simulink model "bike_model_cl"  (R2022b)
settings: Solver=FixedStepAuto  StartTime=0.0  StopTime=20  FixedStep=0.01  RelTol=1e-3
undefined symbols (not defined in the file): gearboxRatio, massTotal_kg, wheelBase_m, wheelBaseRear_m, wheelRadius_m
libraries: autolibshared x3, simulink_extras x2, slpidlib x1
settings Model: Creator=LinF  LastModifiedBy=maxfa
settings SolverCC: ConcurrentTasks=on  PositivePriorityOrder=on
settings OptimizationCC: BlockReduction=off  OptimizeBlockIOStorage=off  BufferReuse=off
settings DebuggingCC: TasksWithSamePriorityMsg=none
settings HardwareCC: ProdBitPerLong=64  ProdLongLongMode=on  ProdHWDeviceType=Intel->x86-64 (Linux 64)
settings RTWCC: Description=Simulink Real-Time  SystemTargetFile=slrealtime.tlc  TemplateMakefile=slrealtime_default_tmf  Toolchain=Simulink Real-Time Toolchain  BuildConfiguration=Faster Runs  CodeExecutionProfiling=on  TargetLang=C++

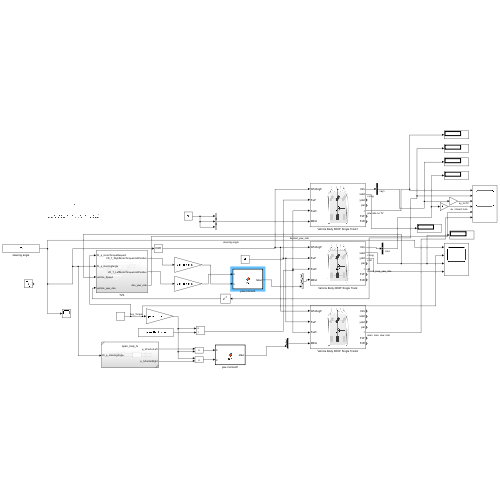
[thumbnail: Simulink's stored preview of the top-level diagram]
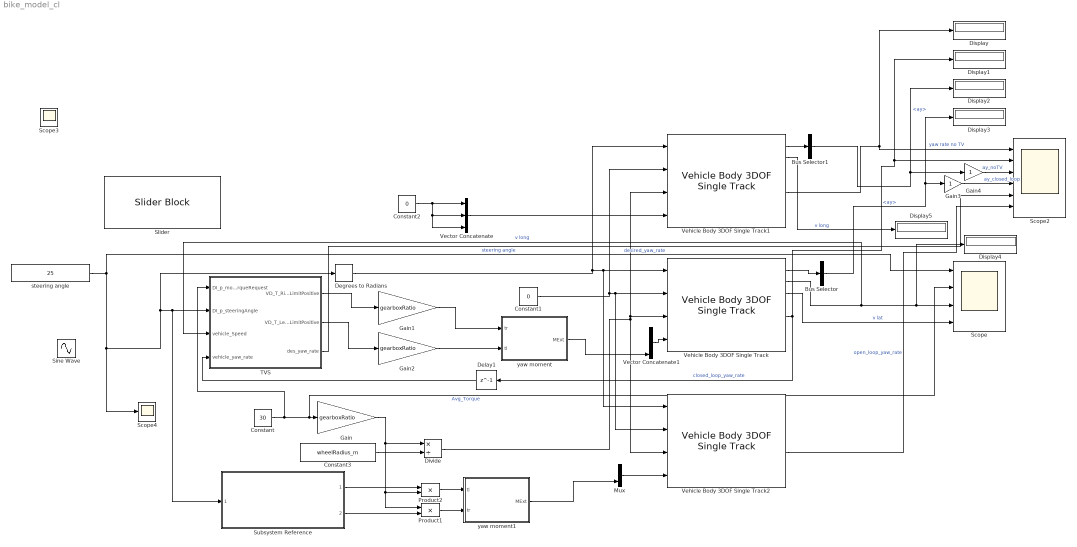
== system bike_model_cl ==
  Bus Selector : BusSelector  OutputSignals=BdyFrm.Cg.Acc.ay
  Bus Selector1 : BusSelector  OutputSignals=BdyFrm.Cg.Acc.ay
  Constant : Constant  Value=30
  Constant1 : Constant  Value=0
  Constant2 : Constant  Value=0
  Constant3 : Constant  Value=wheelRadius_m
  Degrees to Radians : simulink_extras/Transformations/Degrees to Radians
  Delay1 : Delay  DelayLength=1
  Display{,1..5} (6 alike) : Display
  Divide : Product  Inputs=*/
  Gain : Gain  Gain=gearboxRatio
  Gain1 : Gain  Gain=gearboxRatio
  Gain2 : Gain  Gain=gearboxRatio
  Gain3 : Gain
  Gain4 : Gain
  Mux : Mux  Inputs=3
  Product1 : Product
  Product2 : Product
  Scope : Scope  NumInputPorts=4
  Scope2 : Scope  NumInputPorts=6
  Scope4 : Scope
  Sine Wave : Sin  Amplitude=25  SampleTime=0
  Slider : SliderBlock  ScaleMin=-25  ScaleMax=25
  Subsystem Reference : Subsystem  ReferencedSubsystem=open_loop_tv
  TVS : Subsystem
  Vector Concatenate : Concatenate  NumInputs=3
  Vector Concatenate1 : Concatenate  NumInputs=3
  Vehicle Body 3DOF Single Track : autolibshared/Vehicle Body 3DOF Single Track  trackMode=Single (bicycle)  inputMode=External longitudinal forces  frontSteerMode=on  rearSteerMode=off  windMode=off  muMode=off  extFMode=off  extMMode=on  htchFMode=off  htchMMode=off  extXo=off  extpsio=off  extxdoto=off  extro=off  extYo=off  extTamb=off  extydoto=off  aMode=2  NF=2  NR=2  m=massTotal_kg  a=wheelBaseFront_m  b=wheelBaseRear_m  h=cgHeight_m  dh=1  hh=0.2  X_o=0  xdot_o=0  CalphaMode=off  sigmaMode=off  d=0  hl=0  w=[1.4,1.4]  Cy_f=CyFront_N_per_Rad  Cy_r=CyRear_N_per_Rad  sigma_f=.1  sigma_r=.1  alpha_f_brk=[-.1 .1]  Cy_f_data=[-9e3 9e3]  alpha_r_brk=[-.1 .1]  Cy_r_data=[-9e3 9e3]  Y_o=0  ydot_o=0  Izz=yawInertia_kg_per_mSqrd  psi_o=0  r_o=0  Af=dragArea_mSqrd  Cd=Cd  Cl=Cl  Cpm=.1  beta_w=[0 0.01:0.01:0.3]  Cs=[0 0.01:0.01:0.3]  Cym=[0 1e-6:0.01:0.3]  Pabs=101325  Tair=273  g=9.81  mu=1  xdot_tol=.01  Fznom=5000  Fxtire_sat=7e4  Fytire_sat=7e4  longOff=0  latOff=0  vertOff=0  wrapAng=off
  Vehicle Body 3DOF Single Track1 : autolibshared/Vehicle Body 3DOF Single Track  trackMode=Single (bicycle)  inputMode=External longitudinal forces  frontSteerMode=on  rearSteerMode=off  windMode=off  muMode=off  extFMode=off  extMMode=on  htchFMode=off  htchMMode=off  extXo=off  extpsio=off  extxdoto=off  extro=off  extYo=off  extTamb=off  extydoto=off  aMode=2  NF=2  NR=2  m=massTotal_kg  a=wheelBaseFront_m  b=wheelBaseRear_m  h=cgHeight_m  dh=1  hh=0.2  X_o=0  xdot_o=0  CalphaMode=off  sigmaMode=off  d=0  hl=0  w=[1.4,1.4]  Cy_f=CyFront_N_per_Rad  Cy_r=CyRear_N_per_Rad  sigma_f=.1  sigma_r=.1  alpha_f_brk=[-.1 .1]  Cy_f_data=[-9e3 9e3]  alpha_r_brk=[-.1 .1]  Cy_r_data=[-9e3 9e3]  Y_o=0  ydot_o=0  Izz=yawInertia_kg_per_mSqrd  psi_o=0  r_o=0  Af=dragArea_mSqrd  Cd=Cd  Cl=Cl  Cpm=.1  beta_w=[0 0.01:0.01:0.3]  Cs=[0 0.01:0.01:0.3]  Cym=[0 1e-6:0.01:0.3]  Pabs=101325  Tair=273  g=9.81  mu=1  xdot_tol=.01  Fznom=5000  Fxtire_sat=7e4  Fytire_sat=7e4  longOff=0  latOff=0  vertOff=0  wrapAng=off
  Vehicle Body 3DOF Single Track2 : autolibshared/Vehicle Body 3DOF Single Track  trackMode=Single (bicycle)  inputMode=External longitudinal forces  frontSteerMode=on  rearSteerMode=off  windMode=off  muMode=off  extFMode=off  extMMode=on  htchFMode=off  htchMMode=off  extXo=off  extpsio=off  extxdoto=off  extro=off  extYo=off  extTamb=off  extydoto=off  aMode=2  NF=2  NR=2  m=massTotal_kg  a=wheelBaseFront_m  b=wheelBaseRear_m  h=cgHeight_m  dh=1  hh=0.2  X_o=0  xdot_o=0  CalphaMode=off  sigmaMode=off  d=0  hl=0  w=[1.4,1.4]  Cy_f=CyFront_N_per_Rad  Cy_r=CyRear_N_per_Rad  sigma_f=.1  sigma_r=.1  alpha_f_brk=[-.1 .1]  Cy_f_data=[-9e3 9e3]  alpha_r_brk=[-.1 .1]  Cy_r_data=[-9e3 9e3]  Y_o=0  ydot_o=0  Izz=yawInertia_kg_per_mSqrd  psi_o=0  r_o=0  Af=dragArea_mSqrd  Cd=Cd  Cl=Cl  Cpm=.1  beta_w=[0 0.01:0.01:0.3]  Cs=[0 0.01:0.01:0.3]  Cym=[0 1e-6:0.01:0.3]  Pabs=101325  Tair=273  g=9.81  mu=1  xdot_tol=.01  Fznom=5000  Fxtire_sat=7e4  Fytire_sat=7e4  longOff=0  latOff=0  vertOff=0  wrapAng=off
  steering angle : Constant  Value=25
  yaw moment : MATLAB Function  TreatAsAtomicUnit=on
  yaw moment1 : MATLAB Function  TreatAsAtomicUnit=on
  Scope3 : Scope
  wires:
  Vehicle Body 3DOF Single Track/1 -> Bus Selector/1
  Vehicle Body 3DOF Single Track/3 -> Scope/4  "v lat"
  Vehicle Body 3DOF Single Track/2 -> TVS/3(vehicle_Speed), Display4/1, Scope/3  "v long"
  Vehicle Body 3DOF Single Track/5 -> Scope2/2, Display1/1, Delay1/1  "closed_loop_yaw_rate"
  Constant/1 -> TVS/1(DI_p_motorTorqueRequest), Scope/2, Gain/1  "Avg_Torque"
  Degrees to Radians/1 -> Vehicle Body 3DOF Single Track2/1, Vehicle Body 3DOF Single Track/1, Vehicle Body 3DOF Single Track1/1
  yaw moment/1(MExt) -> Vector Concatenate1/3
  steering angle/1 -> Scope/1, Scope4/1, Degrees to Radians/1, Subsystem Reference/1, TVS/2(DI_p_steeringAngle)  "steering angle"
  Vector Concatenate/1 -> Vehicle Body 3DOF Single Track1/4
  Vehicle Body 3DOF Single Track1/5 -> Display/1, Scope2/1  "yaw rate no TV"
  Constant2/1 -> Vector Concatenate/3, Vector Concatenate/2, Vector Concatenate/1
  Constant1/1 -> Vehicle Body 3DOF Single Track2/2, Vehicle Body 3DOF Single Track/2, Vehicle Body 3DOF Single Track1/2
  Constant3/1 -> Divide/2
  Divide/1 -> Vehicle Body 3DOF Single Track/3, Vehicle Body 3DOF Single Track1/3, Vehicle Body 3DOF Single Track2/3
  Vehicle Body 3DOF Single Track1/1 -> Bus Selector1/1
  Bus Selector1/1 -> Display2/1, Gain4/1  "<ay>"
  Bus Selector/1 -> Gain3/1, Display3/1  "<ay>"
  Gain/1 -> Product2/2, Product1/1, Divide/1
  Vehicle Body 3DOF Single Track1/2 -> Display5/1  "v long"
  TVS/1(VD_T_RightMotorTorqueLimitPositive) -> Gain1/1
  TVS/2(VD_T_LeftMotorTorqueLimitPositive) -> Gain2/1
  Delay1/1 -> TVS/4(vehicle_yaw_rate)
  Vector Concatenate1/1 -> Vehicle Body 3DOF Single Track/4
  TVS/3(des_yaw_rate) -> Scope2/5  "desired_yaw_rate"
  Gain1/1 -> yaw moment/1(tr)
  Gain2/1 -> yaw moment/2(tl)
  Product2/1 -> yaw moment1/1(tl)
  Product1/1 -> yaw moment1/2(tr)
  Subsystem Reference/1 -> Product2/1
  Subsystem Reference/2 -> Product1/2
  Vehicle Body 3DOF Single Track2/5 -> Scope2/6  "open_loop_yaw_rate"
  Mux/1 -> Vehicle Body 3DOF Single Track2/4
  yaw moment1/1(MExt) -> Mux/3
  Gain3/1 -> Scope2/4  "ay_closed_loop"
  Gain4/1 -> Scope2/3  "ay_noTV"

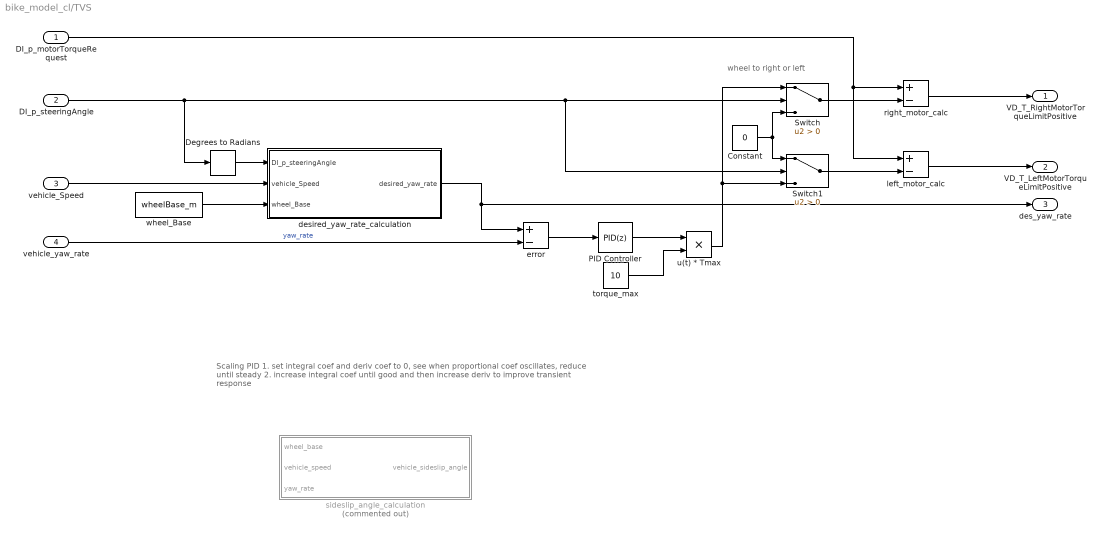
== system bike_model_cl/TVS ==
  note: wheel to right or left
  note: Scaling PID
      | 1. set integral coef and deriv coef to 0, see when proportional coef oscillates, reduce until steady
      | 2. increase integral coef until good and then increase deriv to improve transient response
  DI_p_motorTorqueRequest : Inport
  DI_p_steeringAngle : Inport  Port=2
  vehicle_Speed : Inport  Port=3
  vehicle_yaw_rate : Inport  Port=4
  Constant : Constant  Value=0
  Degrees to Radians : simulink_extras/Transformations/Degrees to Radians
  PID Controller : slpidlib/PID Controller  Controller=PID  Form=Parallel  TimeDomain=Discrete-time  UseExternalTs=off  SampleTime=-1  IntegratorMethod=Forward Euler  FilterMethod=Forward Euler  ControllerParametersSource=internal  P=10  I=5  UseKiTs=off  D=0  N=6.80635582666381  UseFilter=on  TunerSelectOption=Transfer Function Based (PID Tuner App)  InitialConditionSource=internal  InitialConditionForIntegrator=0  InitialConditionForFilter=0  DifferentiatorICPrevScaledInput=0  ExternalReset=none  TrackingMode=off  Kt=1  LimitOutput=off  SatLimitsSource=internal  UpperSaturationLimit=inf  LowerSaturationLimit=-inf  LinearizeAsGain=on  AntiWindupMode=none  Kb=1  LimitIntegrator=off  UpperIntegratorSaturationLimit=inf  LowerIntegratorSaturationLimit=-inf  POutMin=[]  POutMax=[]  IOutMin=[]  IOutMax=[]  DOutMin=[]  DOutMax=[]  NOutMin=[]  NOutMax=[]  SumOutMin=[]  SumOutMax=[]  SaturationOutMin=[]  SaturationOutMax=[]  PParamMin=[]  PParamMax=[]  IParamMin=[]  IParamMax=[]  DParamMin=[]  DParamMax=[]  NParamMin=[]  NParamMax=[]  KbParamMin=[]  KbParamMax=[]  KtParamMin=[]  KtParamMax=[]  KbOutMin=[]  KbOutMax=[]  KtOutMin=[]  KtOutMax=[]  IntegratorOutMin=[]  IntegratorOutMax=[]  FilterOutMin=[]  FilterOutMax=[]  SumI1OutMin=[]  SumI1OutMax=[]  SumI2OutMin=[]  SumI2OutMax=[]  SumI3OutMin=[]  SumI3OutMax=[]  SumI4OutMin=[]  SumI4OutMax=[]  SumDOutMin=[]  SumDOutMax=[]  DifferentiatorOutMin=[]  DifferentiatorOutMax=[]  FilterDiffOutCoefMin=[]  FilterDiffOutCoefMax=[]  ReciprocalOutMin=[]  ReciprocalOutMax=[]  SumDenOutMin=[]  SumDenOutMax=[]  SumNumOutMin=[]  SumNumOutMax=[]  DivideOutMin=[]  DivideOutMax=[]  UdiffTsProdOutMin=[]  UdiffTsProdOutMax=[]  NTsProdOutMin=[]  NTsProdOutMax=[]  UintegralTsProdOutMin=[]  UintegralTsProdOutMax=[]  UngainTsProdOutMin=[]  UngainTsProdOutMax=[]  ClampingZeroOutDataTypeStr=Inherit: Inherit via back propagation  ClampingZeroOutMin=[]  ClampingZeroOutMax=[]  FilterDenConstantOutDataTypeStr=Inherit: Inherit via back propagation  FilterDenConstantOutMin=[]  FilterDenConstantOutMax=[]  PCopyOutDataTypeStr=Inherit: Inherit via back propagation  PCopyOutMin=[]  PCopyOutMax=[]  NCopyOutDataTypeStr=Inherit: Inherit via back propagation  NCopyOutMin=[]  NCopyOutMax=[]  IntegratorContinuousStateAttributes=''  IntegratorStateMustResolveToSignalObject=off  IntegratorRTWStateStorageClass=Auto  FilterContinuousStateAttributes=''  FilterStateMustResolveToSignalObject=off  FilterRTWStateStorageClass=Auto  ParallelPVariant=InternalParameters  IdealPVariant=Disabled  IVariant=InternalParameters  DVariant=InternalParameters  IntegratorVariant=Discrete  SatVariant=Disabled  AWVariant=Passthrough  PCopyVariant=Disabled  TRVariant=Disabled  FdbkBlocksVariant=Forward  IdealPFdbkVariant=Disabled  SatFdbkVariant=Disabled  DerivativeFilterVariant=ForwardEulerFilter  NVariant=InternalParameters  NCopyVariant=Disabled  FilterICVariant=InternalICsFilter  IntegratorICVariant=InternalICs  ExternalResetVariant=Disabled  TRSumVariant=Passthrough  SumFdbkVariant=Disabled  SumVariant=Sum_PID  TsampFilterVariant=InternalTs  TsampNgainVariant=Passthrough  TsampIntegralVariant=Passthrough  ExternalSaturationOutDataTypeStr=Inherit: Same as second input
  Switch : Switch  Criteria=u2 > Threshold  SaturateOnIntegerOverflow=off  InputSameDT=off
  Switch1 : Switch  Criteria=u2 > Threshold  SaturateOnIntegerOverflow=off  InputSameDT=off
  desired_yaw_rate_calculation : Subsystem
  error : Sum  Inputs=+-
  left_motor_calc : Sum  Inputs=+-
  right_motor_calc : Sum  Inputs=+-
  sideslip_angle_calculation : Subsystem  Commented=on
  torque_max : Constant  Value=10
  u(t) * Tmax : Product
  wheel_Base : Constant  Value=wheelBase_m
  VD_T_RightMotorTorqueLimitPositive : Outport
  VD_T_LeftMotorTorqueLimitPositive : Outport  Port=2
  des_yaw_rate : Outport  Port=3
  wires:
  vehicle_yaw_rate/1 -> error/2  "yaw_rate"
  DI_p_steeringAngle/1 -> Degrees to Radians/1, Switch1/2, Switch/2
  vehicle_Speed/1 -> desired_yaw_rate_calculation/2(vehicle_Speed)
  wheel_Base/1 -> desired_yaw_rate_calculation/3(wheel_Base)
  desired_yaw_rate_calculation/1(desired_yaw_rate) -> error/1, des_yaw_rate/1
  error/1 -> PID Controller/1
  DI_p_motorTorqueRequest/1 -> right_motor_calc/1, left_motor_calc/1
  PID Controller/1 -> u(t) * Tmax/1
  torque_max/1 -> u(t) * Tmax/2
  u(t) * Tmax/1 -> Switch/1, Switch1/3
  right_motor_calc/1 -> VD_T_RightMotorTorqueLimitPositive/1
  left_motor_calc/1 -> VD_T_LeftMotorTorqueLimitPositive/1
  Constant/1 -> Switch1/1, Switch/3
  Switch/1 -> right_motor_calc/2
  Switch1/1 -> left_motor_calc/2
  Degrees to Radians/1 -> desired_yaw_rate_calculation/1(DI_p_steeringAngle)

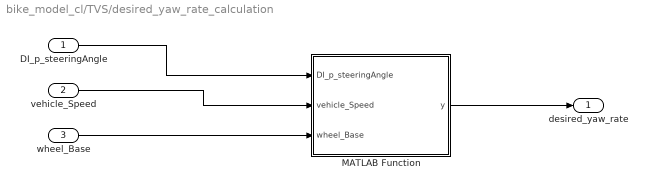
== system bike_model_cl/TVS/desired_yaw_rate_calculation ==
  DI_p_steeringAngle : Inport
  vehicle_Speed : Inport  Port=2
  wheel_Base : Inport  Port=3
  MATLAB Function : MATLAB Function  TreatAsAtomicUnit=on
  desired_yaw_rate : Outport
  wires:
  DI_p_steeringAngle/1 -> MATLAB Function/1(DI_p_steeringAngle)
  vehicle_Speed/1 -> MATLAB Function/2(vehicle_Speed)
  wheel_Base/1 -> MATLAB Function/3(wheel_Base)
  MATLAB Function/1(y) -> desired_yaw_rate/1

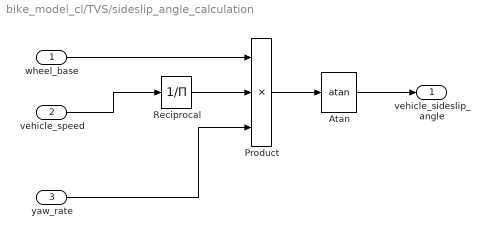
== system bike_model_cl/TVS/sideslip_angle_calculation ==
  wheel_base : Inport
  vehicle_speed : Inport  Port=2
  yaw_rate : Inport  Port=3
  Atan : Trigonometry  Operator=atan
  Product : Product  Inputs=3
  Reciprocal : Product  Inputs=/
  vehicle_sideslip_angle : Outport
  wires:
  Product/1 -> Atan/1
  yaw_rate/1 -> Product/3
  vehicle_speed/1 -> Reciprocal/1
  Atan/1 -> vehicle_sideslip_angle/1
  Reciprocal/1 -> Product/2
  wheel_base/1 -> Product/1

== matlab function bike_model_cl/yaw moment ==
  data: tr input; tl input; MExt output
function MExt = fcn(tr,tl)

tr = double(tr);
tl = double(tl);


m = (tl/0.203-tr/0.203)*0.5*1.285;
MExt = m;

== matlab function bike_model_cl/TVS/desired_yaw_rate_calculation/MATLAB Function ==
  data: DI_p_steeringAngle input; y output; vehicle_Speed input; wheel_Base input
function y = fcn(DI_p_steeringAngle, vehicle_Speed, wheel_Base)

Kus = 0.0026;

y = vehicle_Speed * DI_p_steeringAngle/ (wheel_Base + Kus * vehicle_Speed^2);

== matlab function bike_model_cl/yaw moment1 ==
  data: tl input; MExt output; tr input
function MExt = fcn(tl,tr)

tl = double(tl);
tr = double(tr);

m = (tl/0.203-tr/0.203)*0.5*1.285;
MExt = m;
